simulink library "Delft_Tyre_sm1glib"  (Simulink 6.4)
libraries: mblibv1 x14
settings Model: Creator=kozlowskimk  LastModifiedBy=hofstadrhmtvd

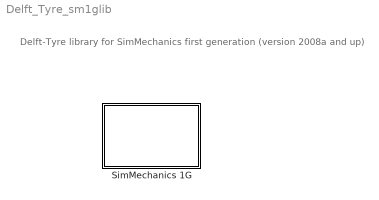
== system Delft_Tyre_sm1glib ==
  note: Delft-Tyre library for SimMechanics
      | first generation (version 2008a and up)
  SimMechanics 1G : Subsystem

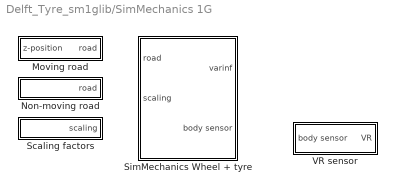
== system Delft_Tyre_sm1glib/SimMechanics 1G ==
  Moving road : Subsystem  Tag=Moving road  mask{response_time=0.05}
      mask prompts: response_time "response time [s]"
  Non-moving road : Subsystem  Tag=Non-moving road  mask{dummy=off}
  Scaling factors : Subsystem  Tag=Scaling factors  mask{LMUX=1, LKX=1, LMUY=1, LKY=1, LKYC=1, LTR=1, LKZC=1}
      mask prompts: LMUX "longitudinal friction"; LKX "longitudinal slip stiffness"; LMUY "lateral fiction"; LKY "cornering stiffness"; LKYC "camber stiffness"; LTR "pneumatic trail"; LKZC "camber torque stiffness"
  SimMechanics Wheel + tyre : Subsystem  Tag=SimMechanics Wheel + tyre  mask(SimMechanics_tyre){idtyre=1, inertia=[10 1 2], tpfname=, rdfname='', side_mode=(1xxx) left, cnt_mode=(x1xx) smooth road, dyn_mode=(xx0x) steady-state, mf_mode=(xxx0) none, use_mode=1e8, disp_debug=off}
      mask prompts: idtyre "Tyre ID [integer]"; inertia "Rim inertia [3x real] mass (kg) Ixx Iyy (kgm2)"; tpfname "Tyre properties [string or struct]"; rdfname "Road data file [string]"; side_mode "Tyre side            :"; cnt_mode "Contact method :"; dyn_mode "Dynamics           :"; mf_mode "Slip forces          :"; use_mode "Optional: use mode (overrides pop-up) [integer]"; disp_debug "Display debug messages"
      mask help:
      | Wheel + tyre model to be used in combination with the SimMechanics multibody toolbox.
      |
      | Tyre model version: MF-Tyre/MF-Swift 6.2
      | © 1996-2013 TNO, Helmond, The Netherlands
      mask init:
      | % initialize parameters
      | % (required to overcome a bug in MATLAB 2006a: errors in a mask are not displayed,
      | %  and simulation is not ended. This check is carried out in s-function 
      | %  'chech_inertia_parameters' in the subsystem)
      | radius     = 1;
      | width      = 1;
      | belt_mass  = 1;
      | belt_Ixx   = 1;
      | belt_Iyy   = 1;
      | tyre_mass  = 1;
      | tyre_Ixx   = 1;
      | tyre_Iyy   = 1;
      | mass = 1;
      | Imat = [1 0 0; 0 1 0; 0 0 1];
      | 
      | % switch between tpf file or struct
      | if ischar(tpfname)
      |     typarr=zeros(300,1);
      |     tpfname_dummy=tpfname;
      |     if ~exist(tpfname_dummy)
      |         error('Tyre property file does not exist')
      |     end
      | elseif isstruct(tpfname)
      |     typarr=tno_tpf_struct2array(tpfname,idtyre);
      |     tpfname_dummy='';
      | else
      |     typarr=zeros(300,1);
      |     tpfname_dummy='';
      |     error(['Mask parameter ''Tyre property file'' should be supplied as string or structure for tyre ' num2str(idtyre)])
      | end
      | if ~exist(rdfname) && ~strcmp(rdfname,'')
      |     error('Road data file does not exist')
      | end
      | 
      | %initialisation script for SimMechanics
      | idroad=1;
      | 
      | %rim inertia as specified by the user in the GUI
      | rim_mass = inertia(1);
      | rim_Ixx  = inertia(2);
      | rim_Iyy  = inertia(3);
      | 
      | % check the use_mode of the model
      | if (abs(use_mode) > 4535 )
      |   iswtch=1000*side_mode+100*cnt_mode+10*(dyn_mode-1)+(mf_mode-1);
      | else
      |   iswtch=use_mode;
      | end
      | 
      | %get tyre inertia parameters from the tyre property file
      | if ischar(tpfname)
      |     [x,typarr]=dteval(tpfname_dummy,[1 2 3 4 5 6],1);
      | end
      | radius     = typarr(7);
      | width      = typarr(8);
      | belt_mass  = typarr(164);
      | belt_Ixx   = typarr(195);
      | belt_Iyy   = typarr(162);
      | tyre_mass  = typarr(190);
      | tyre_Ixx   = typarr(191);
      | tyre_Iyy   = typarr(192);
      | 
      | % display the use_mode of the model
      | if (disp_debug) disp(['Delft-Tyre ' num2str(idtyre) ' -> use_mode=' num2str(iswtch) ]); end
      | 
      | % check and calculate inertia of the rim_body
      | if  ( rim_mass <= 0 | rim_Ixx <= 0 | rim_Iyy <= 0 | tyre_mass <= 0 | tyre_Ixx <= 0 | tyre_Iyy <= 0 | belt_mass <= 0 | belt_Ixx <= 0 | belt_Iyy <= 0 )
      |   error('initialisation calculation results in a negative mass and/or inertia!') 
      |   disp_debug=1;
      | end
      | if  ( tyre_mass <= belt_mass | tyre_Ixx <= belt_Ixx | tyre_Iyy <= belt_Iyy  )
      |   error('initialisation calculation error: tyre belt mass/inertia > tyre mass/inertia!') 
      |   disp_debug=1;
      | end
      | 
      | if (disp_debug) 
      |   msg=[' wheel mass = ',num2str(rim_mass+tyre_mass),' kg'];
      |   disp(msg);
      |   msg=[' wheel Ixx  = ',num2str(rim_Ixx+tyre_Ixx),' kgm2'];
      |   disp(msg);
      |   msg=[' wheel Iyy  = ',num2str(rim_Iyy+tyre_Iyy),' kgm2'];
      |   disp(msg);
      |   msg=[' tyre mass  = ',num2str(tyre_mass),' kg (belt mass = ',num2str(belt_mass),' kg)' ];
      |   disp(msg);
      |   msg=[' tyre Ixx   = ',num2str(tyre_Ixx) ,' kgm2 (belt Ixx  = ',num2str(belt_Ixx) ,' kgm2)'];
      |   disp(msg);
      |   msg=[' tyre Iyy   = ',num2str(tyre_Iyy) ,' kgm2 (belt Iyy  = ',num2str(belt_Iyy) ,' kgm2)'];
      |   disp(msg);
      | end
      | 
      | % calculate the mass of the wheelbody in the MBS environment 
      | %   normally           : rim + tyre
      | %   rigid ring dynamics: rim + part of tyre (and separate rigid body inside tyre model)
      | dynmod=iswtch-100*floor(iswtch/100);
      | if (dynmod/10 >= 3) 
      |   %rigid ring dynamics switched on
      |   wheelbody_mass = rim_mass + tyre_mass - belt_mass;
      |   wheelbody_Ixx  = rim_Ixx  + tyre_Ixx  - belt_Ixx;
      |   wheelbody_Iyy  = rim_Iyy  + tyre_Iyy  - belt_Iyy;
      | else
      |   %rigid ring dynamics switched off
      |   wheelbody_mass = rim_mass + tyre_mass;
      |   wheelbody_Ixx  = rim_Ixx  + tyre_Ixx;
      |   wheelbody_Iyy  = rim_Iyy  + tyre_Iyy;
      | end
      | 
      | mass = wheelbody_mass;
      | Imat = [wheelbody_Ixx 0 0; 0 wheelbody_Iyy 0; 0 0 wheelbody_Ixx];
      mask Help: eval('DTOpenHelp(506)')
      mask StyleString: edit,edit,edit,edit,popup((1xxx) left|(2xxx) right|(3xxx) symmetric),popup((x1xx) smooth road|(x2xx) smooth road (motorcycle: circular cross section)|(x3xx) moving road|(x4xx) 2D short wavelength road contact|(x5xx) 3D short wavelength road contact),popup((xx0x) steady-state|(xx1x) relaxation behaviour|(xx2x) relaxation behaviour - non-linear|(xx3x) rigid ring|(xx4x) rigid ring + initial statics),popup((xxx0) none|(xxx1) longitudinal|(xxx2) lateral|(xxx3) uncombined|(xxx4) combined|(xxx5) combined+turnslip),edit,checkbox
      mask CallbackString:
      | ||||promtstr = get_param(gcb,'MaskPromptString');
      | index = find(double(promtstr)==124);
      | maskval = get_param(gcb,'MaskValues');
      | new_mode = [maskval{5}(2) maskval{6}(3) maskval{7}(4) maskval{8}(5)];
      | newpromtstr = [promtstr(1:index(8)) ['Optional: use mode (overrides pop-up) [current selection: ' new_mode ']'] promtstr(index(9):end)];
      | set_param(gcb,'MaskPromptString',newpromtstr);|promtstr = get_param(gcb,'MaskPromptString');
      | index = find(double(promtstr)==124);
      | maskval = get_param(gcb,'MaskValues');
      | new_mode = [maskval{5}(2) maskval{6}(3) maskval{7}(4) maskval{8}(5)];
      | newpromtstr = [promtstr(1:index(8)) ['Optional: use mode (overrides pop-up) [current selection: ' new_mode ']'] promtstr(index(9):end)];
      | set_param(gcb,'MaskPromptString',newpromtstr);|promtstr = get_param(gcb,'MaskPromptString');
      | index = find(double(promtstr)==124);
      | maskval = get_param(gcb,'MaskValues');
      | new_mode = [maskval{5}(2) maskval{6}(3) maskval{7}(4) maskval{8}(5)];
      | newpromtstr = [promtstr(1:index(8)) ['Optional: use mode (overrides pop-up) [current selection: ' new_mode ']'] promtstr(index(9):end)];
      | set_param(gcb,'MaskPromptString',newpromtstr);|promtstr = get_param(gcb,'MaskPromptString');
      | index = find(double(promtstr)==124);
      | maskval = get_param(gcb,'MaskValues');
      | new_mode = [maskval{5}(2) maskval{6}(3) maskval{7}(4) maskval{8}(5)];
      | newpromtstr = [promtstr(1:index(8)) ['Optional: use mode (overrides pop-up) [current selection: ' new_mode ']'] promtstr(index(9):end)];
      | set_param(gcb,'MaskPromptString',newpromtstr);||
  VR sensor : Subsystem  Tag=VR sensor

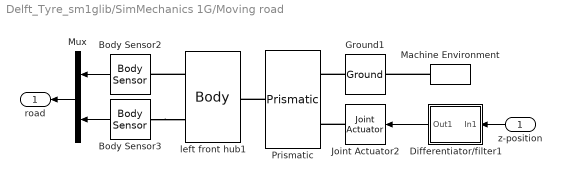
== system Delft_Tyre_sm1glib/SimMechanics 1G/Moving road ==
  z-position : Inport  Orientation=left
  Body Sensor2 : mblibv1/Sensors &  Actuators/Body Sensor  Orientation=left  DialogController=MECH.DynMechDlgSource  SystemSampleTime=-1  PhysicalDomain=Mechanical  PortType=blob  Muxed=on  Pose=on  Angle=on  AngleUnits=deg  ArcVelocity=off  ArcVelocityUnits=rad/s  ArcAcceleration=off  ArcAccelerationUnits=deg/s^2  CoordPosition=on  CoordPositionUnits=m  Velocity=off  VelocityUnits=m/s  Acceleration=off  AccelerationUnits=m/s^2  Quaternion=on  QuaternionDT=off  QuaternionDDT=off  QuaternionUnits=off  OutputVector=[ 3 9 ]  ActiveIO=off  Width=12  DialogClass=MechanicalSensorBlock  ReferenceFrame=Absolute (World)
  Body Sensor3 : mblibv1/Sensors &  Actuators/Body Sensor  Orientation=left  DialogController=MECH.DynMechDlgSource  SystemSampleTime=-1  PhysicalDomain=Mechanical  PortType=blob  Muxed=on  Pose=off  Angle=on  AngleUnits=deg  ArcVelocity=on  ArcVelocityUnits=rad/s  ArcAcceleration=off  ArcAccelerationUnits=deg/s^2  CoordPosition=off  CoordPositionUnits=m  Velocity=on  VelocityUnits=m/s  Acceleration=off  AccelerationUnits=m/s^2  Quaternion=on  QuaternionDT=off  QuaternionDDT=off  QuaternionUnits=off  OutputVector=[ 3 3 ]  ActiveIO=off  Width=6  DialogClass=MechanicalSensorBlock  ReferenceFrame=Absolute (World)
  Differentiator/filter1 : Subsystem  Orientation=left  mask{ts=response_time}
      mask prompts: ts "response_time"
      mask init:
      | c=(3*pi/ts)^2;
  Ground1 : mblibv1/Bodies/Ground  Orientation=left  DialogController=MECH.DynMechDlgSource  SystemSampleTime=-1  LeftPortType=env  RightPortType=workingframe  PhysicalDomain=Mechanical  DialogClass=GroundBlock  CoordPosition=[0 -0.80 0]  CoordPositionUnits=m  StateVectorMgrId=-1  MachineId=[0 0]  ShowEnvPort=on
  Joint Actuator2 : mblibv1/Sensors &  Actuators/Joint Actuator  Orientation=left  DialogController=MECH.DynMechDlgSource  SystemSampleTime=-1  PhysicalDomain=Mechanical  PortType=blob  ActuationStyle=Motion  AngleUnits=deg  ArcVelocityUnits=deg/s  ArcAccelerationUnits=deg/s^2  CoordPositionUnits=m  VelocityUnits=m/s  AccelerationUnits=m/s^2  ForceUnits=N  TorqueUnits=N-m  ActiveIO=off  Width=3  DialogClass=MechanicalActuatorBlock  Primitive=P1  ReferenceFrame=Absolute (INERTIAL)
  Machine Environment : mblibv1/Bodies/Machine Environment  Tag=Factory ground  Orientation=left  DialogController=MECH.DialogSource  SystemSampleTime=-1  PortType=env  PhysicalDomain=Mechanical  DialogTemplateClass=MECH.MachineEnvironment  SyncWhenCopied=off  Gravity=[0 0 -10]  GravityUnits=m/s^2  GravityAsSignal=off  Dimensionality=Auto-detect  AnalysisType=Forward dynamics  LinearAssemblyTolerance=1e-3  LinearAssemblyToleranceUnits=m  AngularAssemblyTolerance=1e-3  AngularAssemblyToleranceUnits=rad  ConstraintSolverType=Stabilizing  ConstraintRelTolerance=1e-4  ConstraintAbsTolerance=1e-4  UseRobustSingularityHandling=off  RedundancyAnalysisToleranceType=Automatically select tolerance  RedundancyAnalysisTolerance=1e-14  StatePerturbationType=Fixed  PerturbationSize=1e-5  VisualizeMachine=off
  Mux : Mux  Orientation=left  Inputs=2
  Prismatic : mblibv1/Joints/Prismatic  Orientation=left  DialogController=MECH.DynMechDlgSource  PhysicalDomain=mechanical  SubClassName=Unknown  LeftPortType=blob  RightPortType=blob  LConnTagsString=__newl0|SA1  RConnTagsString=__newr0  NumSAPorts=1  CutJoint=off  MarkAsCut=off  Primitives=prismatic  PrimitiveProps=P1$WORLD$[0 0 1]$prismatic  DialogClass=JointBlock  P1Axis=[0 0 1]
  left front hub1 : mblibv1/Bodies/Body  Orientation=left  DialogController=MECH.DynMechDlgSource  PhysicalDomain=mechanical  SubClassName=Unknown  LeftPortType=workingframe  RightPortType=workingframe  LConnTagsString=CS1  RConnTagsString=CS2|CS3  DialogClass=MechanicalBodyBlock  Mass=1  MassUnits=kg  InertiaUnits=kg*m^2  Inertia=eye(3)  Shape=Cylinder  ShapeDims=[1 1]  ShapeUnits=m  ShapeUse=false  Density=1  DensityUnits=kg/m^3  DensityUse=false  GraphicsMode=1  BodyColor=[0.5 0.5 0.5]  AttachedToCS=1  CG=Left$CG$[0 0 0]$CS1$CS1$m$[0 0 0]$Euler X-Y-Z$deg$WORLD$false  WorkingFrames=Left$CS1$[0 0 0]$ADJOINING$ADJOINING$m$[0 0 0]$Euler X-Y-Z$deg$WORLD$true#Right$CS2$[0 0 0]$CS1$CS1$m$[0 0 0]$Euler X-Y-Z$deg$WORLD$true#Right$CS3$[0 0 0]$CS1$CS1$m$[0 0 0]$Euler X-Y-Z$deg$WORLD$true  CGPos=[0 0 0]  CGRot=[0 0 0]  CS0Pos=[]  CS0Rot=[]  CS1Pos=[0 0 0]  CS1Rot=[0 0 0]  CS2Pos=[0 0 0]  CS2Rot=[0 0 0]  CS3Pos=[0 0 0]  CS3Rot=[0 0 0]  CS4Pos=[]  CS4Rot=[]  CS5Pos=[]  CS5Rot=[]  CS6Pos=[]  CS6Rot=[]  CS7Pos=[]  CS7Rot=[]  CS8Pos=[]  CS8Rot=[]  CS9Pos=[]  CS9Rot=[]  CS10Pos=[]  CS10Rot=[]  CS11Pos=[]  CS11Rot=[]  CS12Pos=[]  CS12Rot=[]  CS13Pos=[]  CS13Rot=[]  CS14Pos=[]  CS14Rot=[]  CS15Pos=[]  CS15Rot=[]  CS16Pos=[]  CS16Rot=[]  CS17Pos=[]  CS17Rot=[]  CS18Pos=[]  CS18Rot=[]  CS19Pos=[]  CS19Rot=[]  CS20Pos=[]  CS20Rot=[]
  road : Outport  Orientation=left
  wires:
  Body Sensor3/1 -> Mux/2
  Body Sensor2/1 -> Mux/1
  Differentiator/filter1/1(Out1) -> Joint Actuator2/1
  Mux/1 -> road/1
  z-position/1 -> Differentiator/filter1/1(In1)
  connections:
  left front hub1/RConn1 -- Body Sensor2/LConn1
  Body Sensor3/LConn1 -- left front hub1/RConn2
  Ground1/RConn1 -- Prismatic/LConn1
  Joint Actuator2/RConn1 -- Prismatic/LConn2
  Prismatic/RConn1 -- left front hub1/LConn1
  Machine Environment/RConn1 -- Ground1/LConn1

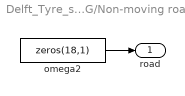
== system Delft_Tyre_sm1glib/SimMechanics 1G/Non-moving road ==
  omega2 : Constant  Value=zeros(18,1)  OutDataType=sfix(16)  ConRadixGroup=Use specified scaling  OutScaling=2^0  SampleTime=inf  FramePeriod=inf
  road : Outport
  wires:
  omega2/1 -> road/1

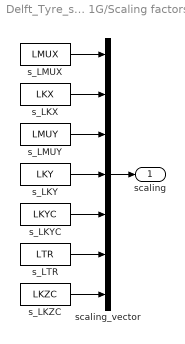
== system Delft_Tyre_sm1glib/SimMechanics 1G/Scaling factors ==
  s_LKX : Constant  Value=LKX  OutDataType=sfix(16)  ConRadixGroup=Use specified scaling  OutScaling=2^0  SampleTime=inf  FramePeriod=inf
  s_LKY : Constant  Value=LKY  OutDataType=sfix(16)  ConRadixGroup=Use specified scaling  OutScaling=2^0  SampleTime=inf  FramePeriod=inf
  s_LKYC : Constant  Value=LKYC  OutDataType=sfix(16)  ConRadixGroup=Use specified scaling  OutScaling=2^0  SampleTime=inf  FramePeriod=inf
  s_LKZC : Constant  Value=LKZC  OutDataType=sfix(16)  ConRadixGroup=Use specified scaling  OutScaling=2^0  SampleTime=inf  FramePeriod=inf
  s_LMUX : Constant  Value=LMUX  OutDataType=sfix(16)  ConRadixGroup=Use specified scaling  OutScaling=2^0  SampleTime=inf  FramePeriod=inf
  s_LMUY : Constant  Value=LMUY  OutDataType=sfix(16)  ConRadixGroup=Use specified scaling  OutScaling=2^0  SampleTime=inf  FramePeriod=inf
  s_LTR : Constant  Value=LTR  OutDataType=sfix(16)  ConRadixGroup=Use specified scaling  OutScaling=2^0  SampleTime=inf  FramePeriod=inf
  scaling_vector : Mux  Inputs=7
  scaling : Outport
  wires:
  s_LMUX/1 -> scaling_vector/1
  s_LKX/1 -> scaling_vector/2
  s_LMUY/1 -> scaling_vector/3
  s_LKY/1 -> scaling_vector/4
  s_LKYC/1 -> scaling_vector/5
  s_LTR/1 -> scaling_vector/6
  s_LKZC/1 -> scaling_vector/7
  scaling_vector/1 -> scaling/1

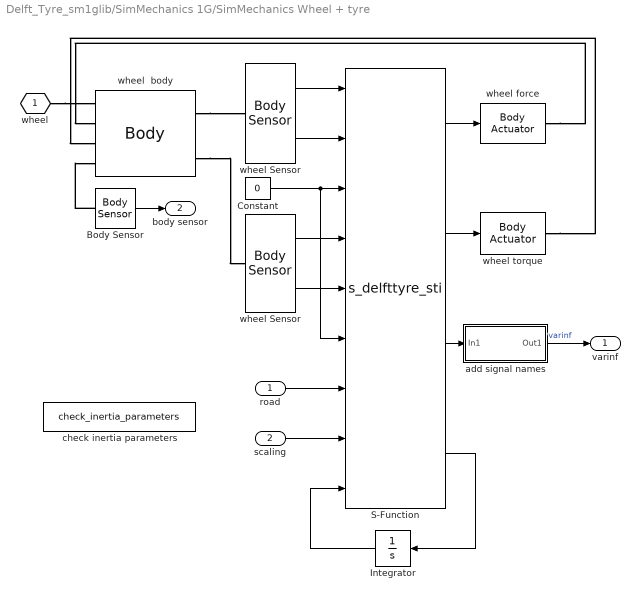
== system Delft_Tyre_sm1glib/SimMechanics 1G/SimMechanics Wheel + tyre ==
  road : Inport
  scaling : Inport  Port=2
  "         wheel force " : mblibv1/Sensors &  Actuators/Body Actuator  DialogController=MECH.DynMechDlgSource  SystemSampleTime=-1  PhysicalDomain=Mechanical  PortType=blob  ActuationStyle=Force  AngleUnits=deg  ArcVelocityUnits=deg/s  ArcAccelerationUnits=deg/s^2  CoordPositionUnits=m  VelocityUnits=m/s  AccelerationUnits=m/s^2  ForceUnits=N  TorqueUnits=N-m  ActiveIO=off  Width=3  DialogClass=MechanicalActuatorBlock  ReferenceFrame=Local (Body CS)  Angle=off  CoordPosition=on  Force=on  Torque=off
  "       wheel torque " : mblibv1/Sensors &  Actuators/Body Actuator  DialogController=MECH.DynMechDlgSource  SystemSampleTime=-1  PhysicalDomain=Mechanical  PortType=blob  ActuationStyle=Force  AngleUnits=deg  ArcVelocityUnits=deg/s  ArcAccelerationUnits=deg/s^2  CoordPositionUnits=m  VelocityUnits=m/s  AccelerationUnits=m/s^2  ForceUnits=N  TorqueUnits=N-m  ActiveIO=off  Width=3  DialogClass=MechanicalActuatorBlock  ReferenceFrame=Local (Body CS)  Angle=off  CoordPosition=on  Force=off  Torque=on
  "      wheel Sensor" : mblibv1/Sensors &  Actuators/Body Sensor  DialogController=MECH.DynMechDlgSource  SystemSampleTime=-1  PhysicalDomain=Mechanical  PortType=blob  Muxed=off  Pose=on  Angle=on  AngleUnits=deg  ArcVelocity=off  ArcVelocityUnits=deg/s  ArcAcceleration=off  ArcAccelerationUnits=deg/s^2  CoordPosition=on  CoordPositionUnits=m  Velocity=off  VelocityUnits=m/s  Acceleration=off  AccelerationUnits=m/s^2  Quaternion=on  QuaternionDT=off  QuaternionDDT=off  QuaternionUnits=off  OutputVector=[ 3 9 ]  ActiveIO=off  Width=12  DialogClass=MechanicalSensorBlock  ReferenceFrame=Absolute (World)
  Body Sensor : mblibv1/Sensors &  Actuators/Body Sensor  DialogController=MECH.DynMechDlgSource  SystemSampleTime=-1  PhysicalDomain=Mechanical  PortType=blob  Muxed=on  Pose=on  Angle=on  AngleUnits=deg  ArcVelocity=off  ArcVelocityUnits=deg/s  ArcAcceleration=off  ArcAccelerationUnits=deg/s^2  CoordPosition=on  CoordPositionUnits=m  Velocity=off  VelocityUnits=m/s  Acceleration=off  AccelerationUnits=m/s^2  Quaternion=on  QuaternionDT=off  QuaternionDDT=off  QuaternionUnits=off  OutputVector=[ 3 9 ]  ActiveIO=off  Width=12  DialogClass=MechanicalSensorBlock  ReferenceFrame=Absolute (World)
  Constant : Constant  Value=0  OutDataType=sfix(16)  ConRadixGroup=Use specified scaling  OutScaling=2^0  SampleTime=inf  FramePeriod=inf
  Integrator : Integrator  Orientation=left  InitialCondition=zeros(1,40)
  S-Function : S-Function  FunctionName=s_delfttyre_sti  Parameters=iswtch idtyre idroad tpfname_dummy rdfname typarr
  add signal names : Subsystem
  check inertia parameters : M-S-Function  Priority=1  FunctionName=check_inertia_parameters  Parameters=tpfname1, rdfname1, typarr1  mask{tpfname1=tpfname_dummy, rdfname1=rdfname, typarr1=typarr}
      mask prompts: tpfname1 "Tyre Property File"; rdfname1 "Road Data File"; typarr1 "typarr"
      mask help: Checks Inertia parameters as calculated in mask
  wheel  body : mblibv1/Bodies/Body  Orientation=left  DialogController=MECH.DynMechDlgSource  PhysicalDomain=mechanical  SubClassName=Unknown  LeftPortType=workingframe  RightPortType=workingframe  LConnTagsString=CS3|CS4  RConnTagsString=CG|CS1|CS2|CS5  DialogClass=MechanicalBodyBlock  Mass=mass  MassUnits=kg  InertiaUnits=kg*m^2  Inertia=Imat  Shape=Cylinder  ShapeDims=[1 1]  ShapeUnits=m  ShapeUse=false  Density=1  DensityUnits=kg/m^3  DensityUse=false  GraphicsMode=1  BodyColor=[0.5 0.5 0.5]  AttachedToCS=1  CG=Right$CG$[0 0 0]$ADJOINING$ADJOINING$m$[0 0 0]$EULER X-Y-Z$deg$ADJOINING$true  WorkingFrames=Right$CS1$[0 0 0]$CG$CG$m$[0 0 0]$EULER X-Y-Z$deg$CG$true#Right$CS2$[0 0 0]$CG$CG$m$[0 0 0]$EULER X-Y-Z$deg$CG$true#Left$CS3$[0 0 0]$CG$CG$m$[0 0 0]$EULER X-Y-Z$deg$CG$true#Left$CS4$[0 0 0]$CG$CG$m$[0 0 0]$EULER X-Y-Z$deg$CG$true#Right$CS5$[0 0 0]$CG$CG$m$[90 0 0]$EULER X-Y-Z$deg$CG$true#Right$CS7$[radius*cos(0) -0.5*width radius*sin(0)]$CG$CG$m$[0 0 0]$EULER X-Y-Z$deg$CG$false#Right$CS17$[radius*cos(0) 0.5*width radius*sin(0)]$CG$CG$m$[0 0 0]$EULER X-Y-Z$deg$CG$false#Right$CS8$[radius*cos(0.2*pi) -0.5*width radius*sin(0.2*pi)]$CG$CG$m$[0 0 0]$EULER X-Y-Z$deg$CG$false#Right$CS18$[radius*cos(0.2*pi) 0.5*width radius*sin(0.2*pi)]$CG$CG$m$[0 0 0]$EULER X-Y-Z$deg$CG$false#Right$CS9$[radius*cos(0.4*pi) -0.5*width radius*sin(0.4*pi)]$CG$CG$m$[0 0 0]$EULER X-Y-Z$deg$CG$false#Right$CS19$[radius*cos(0.4*pi) 0.5*width radius*sin(0.4*pi)]$CG$CG$m$[0 0 0]$EULER X-Y-Z$deg$CG$false#Right$CS10$[radius*cos(0.6*pi) -0.5*width radius*sin(0.6*pi)]$CG$CG$m$[0 0 0]$EULER X-Y-Z$deg$CG$false#Right$CS20$[radius*cos(0.6*pi) 0.5*width radius*sin(0.6*pi)]$CG$CG$m$[0 0 0]$EULER X-Y-Z$deg$CG$false#Right$CS11$[radius*cos(0.8*pi) -0.5*width radius*sin(0.8*pi)]$CG$CG$m$[0 0 0]$EULER X-Y-Z$deg$CG$false#Right$CS21$[radius*cos(0.8*pi) 0.5*width radius*sin(0.8*pi)]$CG$CG$m$[0 0 0]$EULER X-Y-Z$deg$CG$false#Right$CS12$[radius*cos(1.0*pi) -0.5*width radius*sin(1.0*pi)]$CG$CG$m$[0 0 0]$EULER X-Y-Z$deg$CG$false#Right$CS22$[radius*cos(1.0*pi) 0.5*width radius*sin(1.0*pi)]$CG$CG$m$[0 0 0]$EULER X-Y-Z$deg$CG$false#Right$CS13$[radius*cos(1.2*pi) -0.5*width radius*sin(1.2*pi)]$CG$CG$m$[0 0 0]$EULER X-Y-Z$deg$CG$false#Right$CS23$[radius*cos(1.2*pi) 0.5*width radius*sin(1.2*pi)]$CG$CG$m$[0 0 0]$EULER X-Y-Z$deg$CG$false#Right$CS14$[radius*cos(1.4*pi) -0.5*width radius*sin(1.4*pi)]$CG$CG$m$[0 0 0]$EULER X-Y-Z$deg$CG$false#Right$CS24$[radius*cos(1.4*pi) 0.5*width radius*sin(1.4*pi)]$CG$CG$m$[0 0 0]$EULER X-Y-Z$deg$CG$false#Right$CS15$[radius*cos(1.6*pi) -0.5*width radius*sin(1.6*pi)]$CG$CG$m$[0 0 0]$EULER X-Y-Z$deg$CG$false#Right$CS25$[radius*cos(1.6*pi) 0.5*width radius*sin(1.6*pi)]$CG$CG$m$[0 0 0]$EULER X-Y-Z$deg$CG$false#Right$CS16$[radius*cos(1.8*pi) -0.5*width radius*sin(1.8*pi)]$CG$CG$m$[0 0 0]$EULER X-Y-Z$deg$CG$false#Right$CS26$[radius*cos(1.8*pi) 0.5*width radius*sin(1.8*pi)]$CG$CG$m$[0 0 0]$EULER X-Y-Z$deg$CG$false  CGPos=[0 0 0]  CGRot=[0 0 0]  CS0Pos=[]  CS0Rot=[]  CS1Pos=[0 0 0]  CS1Rot=[0 0 0]  CS2Pos=[0 0 0]  CS2Rot=[0 0 0]  CS3Pos=[0 0 0]  CS3Rot=[0 0 0]  CS4Pos=[0 0 0]  CS4Rot=[0 0 0]  CS5Pos=[0 0 0]  CS5Rot=[90 0 0]  CS6Pos=[]  CS6Rot=[]  CS7Pos=[radius*cos(0) -0.5*width radius*sin(0)]  CS7Rot=[0 0 0]  CS8Pos=[radius*cos(0.2*pi) -0.5*width radius*sin(0.2*pi)]  CS8Rot=[0 0 0]  CS9Pos=[radius*cos(0.4*pi) -0.5*width radius*sin(0.4*pi)]  CS9Rot=[0 0 0]  CS10Pos=[radius*cos(0.6*pi) -0.5*width radius*sin(0.6*pi)]  CS10Rot=[0 0 0]  CS11Pos=[radius*cos(0.8*pi) -0.5*width radius*sin(0.8*pi)]  CS11Rot=[0 0 0]  CS12Pos=[radius*cos(1.0*pi) -0.5*width radius*sin(1.0*pi)]  CS12Rot=[0 0 0]  CS13Pos=[radius*cos(1.2*pi) -0.5*width radius*sin(1.2*pi)]  CS13Rot=[0 0 0]  CS14Pos=[radius*cos(1.4*pi) -0.5*width radius*sin(1.4*pi)]  CS14Rot=[0 0 0]  CS15Pos=[radius*cos(1.6*pi) -0.5*width radius*sin(1.6*pi)]  CS15Rot=[0 0 0]  CS16Pos=[radius*cos(1.8*pi) -0.5*width radius*sin(1.8*pi)]  CS16Rot=[0 0 0]  CS17Pos=[radius*cos(0) 0.5*width radius*sin(0)]  CS17Rot=[0 0 0]  CS18Pos=[radius*cos(0.2*pi) 0.5*width radius*sin(0.2*pi)]  CS18Rot=[0 0 0]  CS19Pos=[radius*cos(0.4*pi) 0.5*width radius*sin(0.4*pi)]  CS19Rot=[0 0 0]  CS20Pos=[radius*cos(0.6*pi) 0.5*width radius*sin(0.6*pi)]  CS20Rot=[0 0 0]
  wheel Sensor : mblibv1/Sensors &  Actuators/Body Sensor  DialogController=MECH.DynMechDlgSource  SystemSampleTime=-1  PhysicalDomain=Mechanical  PortType=blob  Muxed=off  Pose=off  Angle=on  AngleUnits=deg  ArcVelocity=on  ArcVelocityUnits=rad/s  ArcAcceleration=off  ArcAccelerationUnits=deg/s^2  CoordPosition=off  CoordPositionUnits=m  Velocity=on  VelocityUnits=m/s  Acceleration=off  AccelerationUnits=m/s^2  Quaternion=on  QuaternionDT=off  QuaternionDDT=off  QuaternionUnits=off  OutputVector=[ 3 3 ]  ActiveIO=off  Width=6  DialogClass=MechanicalSensorBlock  ReferenceFrame=Local (Body CS)
  wheel : PMIOPort  Port=1  Side=Left
  varinf : Outport
  body sensor : Outport  Port=2
  wires:
  wheel Sensor/2 -> S-Function/5
  wheel Sensor/1 -> S-Function/4
  "      wheel Sensor"/2 -> S-Function/2
  "      wheel Sensor"/1 -> S-Function/1
  S-Function/2 -> "       wheel torque "/1
  S-Function/1 -> "         wheel force "/1
  Constant/1 -> S-Function/6, S-Function/3
  add signal names/1(Out1) -> varinf/1  "varinf"
  S-Function/3 -> add signal names/1(In1)
  scaling/1 -> S-Function/8
  Integrator/1 -> S-Function/9
  S-Function/4 -> Integrator/1
  Body Sensor/1 -> body sensor/1
  road/1 -> S-Function/7
  connections:
  wheel/RConn1 -- wheel  body/RConn1
  Body Sensor/LConn1 -- wheel  body/RConn4
  "         wheel force "/RConn1 -- wheel  body/RConn2
  "       wheel torque "/RConn1 -- wheel  body/RConn3
  wheel  body/LConn1 -- "      wheel Sensor"/LConn1
  wheel  body/LConn2 -- wheel Sensor/LConn1

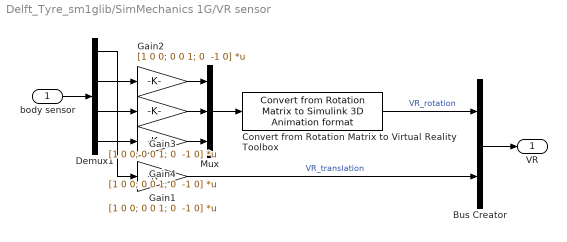
== system Delft_Tyre_sm1glib/SimMechanics 1G/VR sensor ==
  body sensor : Inport  OutDataType=fixdt(1,16,0)  OutScaling=[]
  Bus Creator : BusCreator  Inputs=2
  Convert from Rotation Matrix to Virtual Reality Toolbox : mblibv1/Utilities/Convert from Rotation Matrix to Simulink 3D Animation format  Tag=Pose2VR
  Demux1 : Demux  Outputs=[3 3 3 3]
  Gain{1..4} (4 alike) : Gain  Gain="[1 0 0; 0 0 1; 0  -1 0]"  Multiplication=Matrix(K*u)  ParameterDataType=fixdt(1,16,0)  ParameterScaling=[]  OutDataType=fixdt(1,16,0)  OutScaling=[]  SaturateOnIntegerOverflow=on
  Mux : Mux  Inputs=3
  VR : Outport  OutDataType=fixdt(1,16,0)  OutScaling=[]
  wires:
  Bus Creator/1 -> VR/1
  Demux1/2 -> Gain2/1
  Demux1/3 -> Gain3/1
  Demux1/4 -> Gain4/1
  Mux/1 -> Convert from Rotation Matrix to Virtual Reality Toolbox/1
  Gain2/1 -> Mux/1
  Gain3/1 -> Mux/2
  Gain4/1 -> Mux/3
  Convert from Rotation Matrix to Virtual Reality Toolbox/1 -> Bus Creator/1  "VR_rotation"
  Gain1/1 -> Bus Creator/2  "VR_translation"
  Demux1/1 -> Gain1/1
  body sensor/1 -> Demux1/1

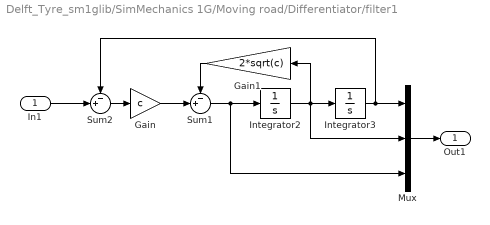
== system Delft_Tyre_sm1glib/SimMechanics 1G/Moving road/Differentiator/filter1 ==
  In1 : Inport
  Gain : Gain  Gain=c  SaturateOnIntegerOverflow=on
  Gain1 : Gain  Orientation=left  Gain=2*sqrt(c)  SaturateOnIntegerOverflow=on
  Integrator2 : Integrator
  Integrator3 : Integrator
  Mux : Mux  Inputs=3
  Sum1 : Sum  Inputs=-+|  SaturateOnIntegerOverflow=on
  Sum2 : Sum  Inputs=-+|  SaturateOnIntegerOverflow=on
  Out1 : Outport
  wires:
  Integrator2/1 -> Integrator3/1, Mux/2, Gain1/1
  Integrator3/1 -> Mux/1, Sum2/1
  Mux/1 -> Out1/1
  Sum1/1 -> Mux/3, Integrator2/1
  Sum2/1 -> Gain/1
  In1/1 -> Sum2/2
  Gain1/1 -> Sum1/1
  Gain/1 -> Sum1/2

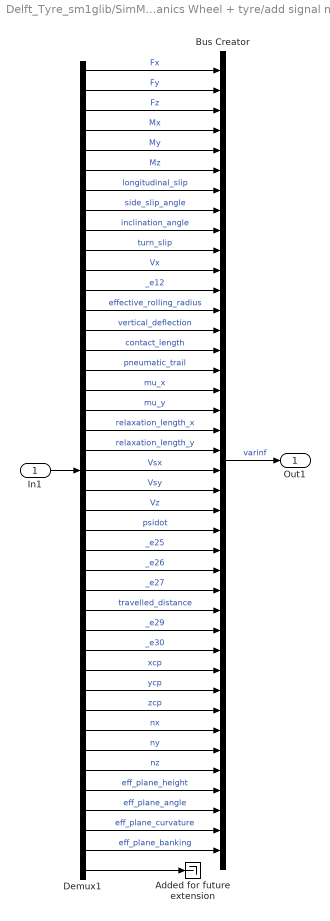
== system Delft_Tyre_sm1glib/SimMechanics 1G/SimMechanics Wheel + tyre/add signal names ==
  In1 : Inport
  Added for future extension : Terminator
  Bus Creator : BusCreator  Inputs=40
  Demux1 : Demux  Outputs=[ones(1,40) -1]
  Out1 : Outport
  wires:
  In1/1 -> Demux1/1
  Bus Creator/1 -> Out1/1  "varinf"
  Demux1/1 -> Bus Creator/1  "Fx"
  Demux1/2 -> Bus Creator/2  "Fy"
  Demux1/3 -> Bus Creator/3  "Fz"
  Demux1/4 -> Bus Creator/4  "Mx"
  Demux1/5 -> Bus Creator/5  "My"
  Demux1/6 -> Bus Creator/6  "Mz"
  Demux1/7 -> Bus Creator/7  "longitudinal_slip"
  Demux1/8 -> Bus Creator/8  "side_slip_angle"
  Demux1/9 -> Bus Creator/9  "inclination_angle"
  Demux1/10 -> Bus Creator/10  "turn_slip"
  Demux1/11 -> Bus Creator/11  "Vx"
  Demux1/12 -> Bus Creator/12  "_e12"
  Demux1/13 -> Bus Creator/13  "effective_rolling_radius"
  Demux1/14 -> Bus Creator/14  "vertical_deflection"
  Demux1/15 -> Bus Creator/15  "contact_length"
  Demux1/16 -> Bus Creator/16  "pneumatic_trail"
  Demux1/17 -> Bus Creator/17  "mu_x"
  Demux1/18 -> Bus Creator/18  "mu_y"
  Demux1/19 -> Bus Creator/19  "relaxation_length_x"
  Demux1/20 -> Bus Creator/20  "relaxation_length_y"
  Demux1/21 -> Bus Creator/21  "Vsx"
  Demux1/22 -> Bus Creator/22  "Vsy"
  Demux1/23 -> Bus Creator/23  "Vz"
  Demux1/24 -> Bus Creator/24  "psidot"
  Demux1/25 -> Bus Creator/25  "_e25"
  Demux1/26 -> Bus Creator/26  "_e26"
  Demux1/27 -> Bus Creator/27  "_e27"
  Demux1/28 -> Bus Creator/28  "travelled_distance"
  Demux1/29 -> Bus Creator/29  "_e29"
  Demux1/30 -> Bus Creator/30  "_e30"
  Demux1/31 -> Bus Creator/31  "xcp"
  Demux1/32 -> Bus Creator/32  "ycp"
  Demux1/33 -> Bus Creator/33  "zcp"
  Demux1/34 -> Bus Creator/34  "nx"
  Demux1/35 -> Bus Creator/35  "ny"
  Demux1/36 -> Bus Creator/36  "nz"
  Demux1/37 -> Bus Creator/37  "eff_plane_height"
  Demux1/38 -> Bus Creator/38  "eff_plane_angle"
  Demux1/39 -> Bus Creator/39  "eff_plane_curvature"
  Demux1/40 -> Bus Creator/40  "eff_plane_banking"
  Demux1/41 -> Added for future extension/1
